simulink model "LQRxSTM"  (R2025b)
settings: Solver=FixedStepDiscrete  StartTime=0.0  StopTime=inf  FixedStep=0.005  RelTol=1e-3
settings Model: Creator=mwali  LastModifiedBy=hassa
settings OptimizationCC: DefaultParameterBehavior=Inlined  UseDivisionForNetSlopeComputation=on  GainParamInheritBuiltInType=on  UseFloatMulNetSlope=on  InlineInvariantSignals=on  PassReuseOutputArgsAs=Individual arguments  ZeroExternalMemoryAtStartup=off  ZeroInternalMemoryAtStartup=off  NoFixptDivByZeroProtection=on  EfficientFloat2IntCast=on  LifeSpan=1  MaxStackSize=512  OptimizeBlockOrder=speed  DifferentSizesBufferReuse=on  EfficientTunableParamExpr=on
settings DebuggingCC: ParameterTunabilityLossMsg=error
settings HardwareCC: ProdBitPerPointer=32.0  ProdBitPerSizeT=32.0  ProdBitPerPtrDiffT=32.0  ProdLargestAtomicInteger=Long  ProdLargestAtomicFloat=Double  ProdWordSize=32.0  ProdLongLongMode=on  ProdHWDeviceType=ARM Compatible->ARM Cortex-M
settings SFSimCC: MATLABDynamicMemAlloc=off
settings RTWCC: SystemTargetFile=ert.tlc  HardwareBoard=STM32H7xx Based (Single-core)  TemplateMakefile=ert_default_tmf  Toolchain=GNU Tools for ARM Embedded Processors  Description=Embedded Coder
settings CodeAppCC: ForceParamTrailComments=on  IgnoreCustomStorageClasses=off  OperatorAnnotations=on  SimulinkDataObjDesc=on  SFDataObjDesc=on  CustomSymbolStrGlobalVar=rt$N$M  CustomSymbolStrType=$N$M  CustomSymbolStrFcn=$N$M$F  CustomSymbolStrMacro=$N$M  InsertBlockDesc=on
settings ERTTargetCC: ExtModeTransport=3.0  ExtModeStaticAlloc=on  ExtModeStaticAllocSize=2048.0  ExtModeMexFile=ext_xcp  ExtModeIntrfLevel=Level2 - Open  ERTFilePackagingFormat=CompactWithDataFile  TargetLangStandard=C99 (ISO)  CodeReplacementLibrary=ARM Cortex-M  IncludeMdlTerminateFcn=off  CombineSignalStateStructs=on  SupportAbsoluteTime=off  SupportComplex=off  SupportNonInlinedSFcns=on

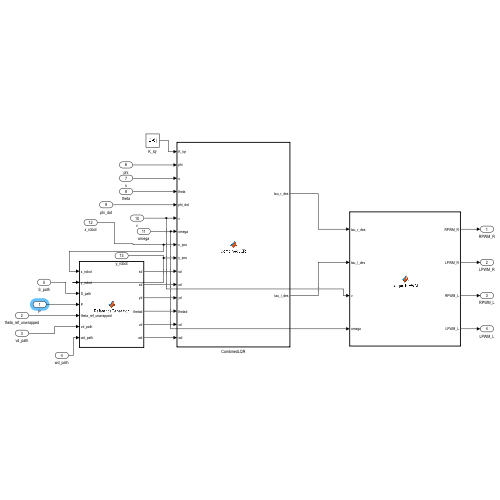
[thumbnail: Simulink's stored preview of the top-level diagram]
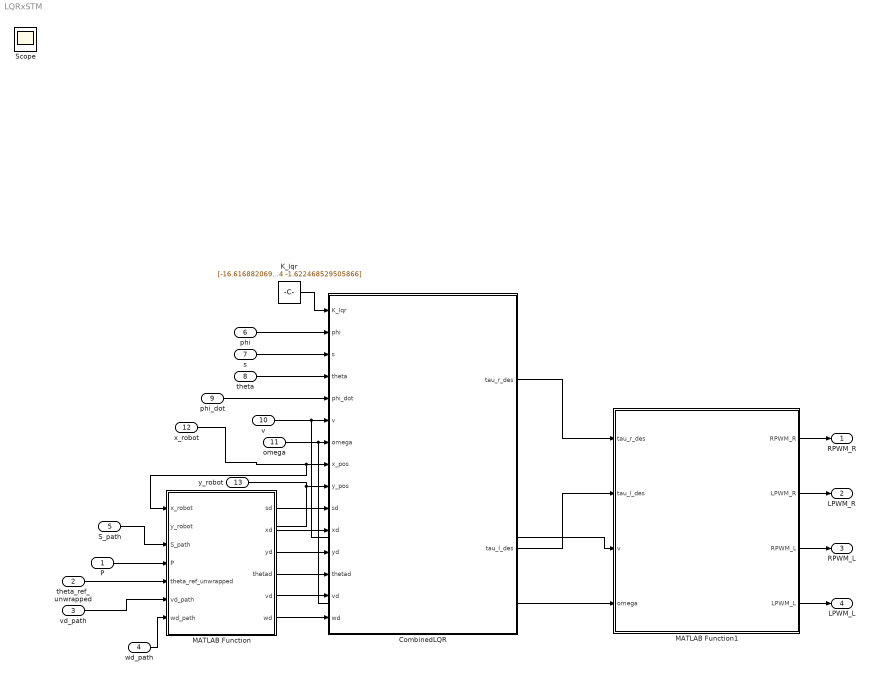
== system LQRxSTM ==
  P : Inport  PortDimensions=[100 2]
  theta_ref_unwrapped : Inport  Port=2  PortDimensions=100
  vd_path : Inport  Port=3  PortDimensions=100
  wd_path : Inport  Port=4  PortDimensions=100
  S_path : Inport  Port=5  PortDimensions=100
  phi : Inport  Port=6
  s : Inport  Port=7
  theta : Inport  Port=8
  phi_dot : Inport  Port=9
  v : Inport  Port=10
  omega : Inport  Port=11
  x_robot : Inport  Port=12
  y_robot : Inport  Port=13
  CombinedLQR : MATLAB Function  TreatAsAtomicUnit=on
  K_lqr : Constant  Value=|
      | [-16.616882069954595	-1.118033988749899	3.162277660168384	-2.938330914554923	-2.061355185548641	1.622468529505869;
      | -16.616882069954599	-1.118033988749900	-3.162277660168376	-2.938330914554922	-2.061355185548644	-1.622468529505866]
  MATLAB Function : MATLAB Function  TreatAsAtomicUnit=on
  MATLAB Function1 : MATLAB Function  TreatAsAtomicUnit=on
  RPWM_R : Outport
  LPWM_R : Outport  Port=2
  RPWM_L : Outport  Port=3
  LPWM_L : Outport  Port=4
  Scope : Scope
      settings: ActiveDisplayYMinimum=-0.34848844243079913  ActiveDisplayYMaximum=2.6945477005962535
  wires:
  MATLAB Function/2(xd) -> CombinedLQR/11(xd)
  phi_dot/1 -> CombinedLQR/5(phi_dot)
  theta/1 -> CombinedLQR/4(theta)
  S_path/1 -> MATLAB Function/3(S_path)
  MATLAB Function/3(yd) -> CombinedLQR/12(yd)
  y_robot/1 -> MATLAB Function/2(y_robot), CombinedLQR/9(y_pos)
  v/1 -> MATLAB Function1/3(v), CombinedLQR/6(v)
  omega/1 -> MATLAB Function1/4(omega), CombinedLQR/7(omega)
  x_robot/1 -> MATLAB Function/1(x_robot), CombinedLQR/8(x_pos)
  s/1 -> CombinedLQR/3(s)
  MATLAB Function1/2(LPWM_R) -> LPWM_R/1
  MATLAB Function1/1(RPWM_R) -> RPWM_R/1
  MATLAB Function/1(sd) -> CombinedLQR/10(sd)
  CombinedLQR/1(tau_r_des) -> MATLAB Function1/1(tau_r_des)
  CombinedLQR/2(tau_l_des) -> MATLAB Function1/2(tau_l_des)
  MATLAB Function/6(wd) -> CombinedLQR/15(wd)
  MATLAB Function/4(thetad) -> CombinedLQR/13(thetad)
  phi/1 -> CombinedLQR/2(phi)
  MATLAB Function/5(vd) -> CombinedLQR/14(vd)
  K_lqr/1 -> CombinedLQR/1(K_lqr)
  MATLAB Function1/3(RPWM_L) -> RPWM_L/1
  MATLAB Function1/4(LPWM_L) -> LPWM_L/1
  P/1 -> MATLAB Function/4(P)
  theta_ref_unwrapped/1 -> MATLAB Function/5(theta_ref_unwrapped)
  vd_path/1 -> MATLAB Function/6(vd_path)
  wd_path/1 -> MATLAB Function/7(wd_path)

== matlab function LQRxSTM/CombinedLQR ==
  settings: updateMethod=DISCRETE
  data: K_lqr input; phi input; s input; theta input; phi_dot input; v input; omega input; x_pos input; y_pos input; sd input; xd input; yd input; thetad input; vd input; wd input; tau_r_des output; tau_l_des output
function [tau_r_des, tau_l_des] = CombinedLQR( ...
    K_lqr, phi, s, theta, phi_dot, v, omega, x_pos, y_pos, ...
    sd, xd, yd, thetad, vd, wd)
%#codegen

% outputs init
tau_r_des  = 0;
tau_l_des  = 0;
ex_out     = 0;
ey_out     = 0;
etheta_out = 0;

% -----------------------------
% 1) Path position error in world frame
% -----------------------------
dx = xd - x_pos;
dy = yd - y_pos;

% -----------------------------
% 2) Error in robot body frame
% ex = forward error
% et = lateral error
% -----------------------------
ex =  cos(theta)*dx + sin(theta)*dy;
ey = -sin(theta)*dx + cos(theta)*dy;

% save for plotting
ex_out = ex;
ey_out = ey;

% -----------------------------
% 3) Heading correction from lateral error
% -----------------------------
k_y = 0.1;                     % tune this if needed
theta_corr_max = deg2rad(20);  % max heading correction

theta_corr = k_y * ey;

if theta_corr > theta_corr_max
    theta_corr = theta_corr_max;
elseif theta_corr < -theta_corr_max
    theta_corr = -theta_corr_max;
end

thetad_corr = thetad + theta_corr;

% -----------------------------
% 4) State error for LQR
% -----------------------------
e = zeros(6,1);
e(1) =phi ;
e(2) = s - sd; 
e(3) = atan2(sin(theta - thetad_corr), cos(theta - thetad_corr));
e(4) = phi_dot;
e(5) = v - vd;
e(6) = omega - wd;

etheta_out = e(3);

% -----------------------------
% 5) LQR control
% -----------------------------
u_des = -K_lqr * e;

tau_r_des = u_des(1);
tau_l_des = u_des(2);

% -----------------------------
% 6) Torque saturation
% -----------------------------
tau_lim = 3; % Changed from 6 to 3

if tau_r_des > tau_lim
    tau_r_des = tau_lim;
elseif tau_r_des < -tau_lim
    tau_r_des = -tau_lim;
end

if tau_l_des > tau_lim
    tau_l_des = tau_lim;
elseif tau_l_des < -tau_lim
    tau_l_des = -tau_lim;
end

== matlab function LQRxSTM/MATLAB Function ==
  data: x_robot input; y_robot input; S_path input; P input; theta_ref_unwrapped input; vd_path input; wd_path input; sd output; xd output; yd output; thetad output; vd output; wd output
function [sd, xd, yd, thetad, vd, wd] = ReferenceGenerator(x_robot, y_robot, S_path, P, theta_ref_unwrapped, vd_path, wd_path)
    N = size(P, 1);

    % 1. Find the nearest discrete node
    min_dist2 = inf;
    k_min = int32(1);
    for k = int32(1) : int32(N)
        dx = P(k, 1) - x_robot;
        dy = P(k, 2) - y_robot;
        d2 = dx*dx + dy*dy;
        if d2 < min_dist2
            min_dist2 = d2;
            k_min = k;
        end
    end

    % 2. Continuous Projection (Fixes the high-frequency torque chattering)
    k_next = min(k_min + int32(1), int32(N));
    k_prev = max(k_min - int32(1), int32(1));

    d2_next = (P(k_next,1)-x_robot)^2 + (P(k_next,2)-y_robot)^2;
    d2_prev = (P(k_prev,1)-x_robot)^2 + (P(k_prev,2)-y_robot)^2;

    if d2_next < d2_prev
        k1 = k_min;
        k2 = k_next;
    else
        k1 = k_prev;
        k2 = k_min;
    end

    if k1 == k2
        alpha = 0.0;
    else
        vx = P(k2,1) - P(k1,1);
        vy = P(k2,2) - P(k1,2);
        L2 = vx*vx + vy*vy;
        if L2 > 1e-6
            rx = x_robot - P(k1,1);
            ry = y_robot - P(k1,2);
            % Orthogonal projection scalar
            alpha = (rx*vx + ry*vy) / L2;
            alpha = max(0.0, min(1.0, alpha));
        else
            alpha = 0.0;
        end
    end

    % 3. Interpolate perfectly smooth references (No Lookahead)
    sd     = (1 - alpha) * S_path(k1) + alpha * S_path(k2);
    xd     = (1 - alpha) * P(k1, 1)   + alpha * P(k2, 1);
    yd     = (1 - alpha) * P(k1, 2)   + alpha * P(k2, 2);
    thetad = (1 - alpha) * theta_ref_unwrapped(k1) + alpha * theta_ref_unwrapped(k2);
    vd     = (1 - alpha) * vd_path(k1) + alpha * vd_path(k2);
    wd     = (1 - alpha) * wd_path(k1) + alpha * wd_path(k2);

    % 4. Safety clamps
    vd_max = 0.3;
    wd_max = 0.334;
    vd = max(0, min(vd, vd_max));
    wd = max(min(wd, wd_max), -wd_max);
end

== matlab function LQRxSTM/MATLAB Function1 ==
  data: tau_r_des input; RPWM_R output; tau_l_des input; v input; omega input; LPWM_R output; RPWM_L output; LPWM_L output
function [RPWM_R, LPWM_R, RPWM_L, LPWM_L] = TorqueToPWM(tau_r_des, tau_l_des, v, omega)
    % --- NFP-42GP-775-EN Motor Parameters ---
    K_t = 0.6746;      % Torque constant (Nm/A)
    K_e = 0.6746;      % Back-EMF constant (V/(rad/s))
    R_res = 0.9796;    % Armature resistance (Ohms)
    V_batt = 24.0;     % Battery voltage (V)
    
    % --- Controller & Robot Parameters ---
    max_pwm = 1000;    % 10-bit timer
    r = 0.060;         % Wheel radius (m)
    d = 0.450;         % Wheelbase (m)
    
    % 1. Estimate wheel speeds (rad/s)
    omega_wheel_r = (v + (omega * d / 2)) / r;
    omega_wheel_l = (v - (omega * d / 2)) / r;

    % 2. Calculate Voltages (V = I*R + Back_EMF)
    v_r = ((tau_r_des / K_t) * R_res) + (K_e * omega_wheel_r);
    v_l = ((tau_l_des / K_t) * R_res) + (K_e * omega_wheel_l);

    % 3. Convert to PWM and Clamp
    pwm_r = round((v_r / V_batt) * max_pwm);
    pwm_l = round((v_l / V_batt) * max_pwm);
    
    % Clamping logic
    pwm_r = max(min(pwm_r, max_pwm), -max_pwm);
    pwm_l = max(min(pwm_l, max_pwm), -max_pwm);

    if pwm_r >= 0
        RPWM_R = pwm_r;
        LPWM_R = 0;
    else
        RPWM_R = 0;
        LPWM_R = abs(pwm_r); 
    end

    if pwm_l >= 0
        RPWM_L = pwm_l;
        LPWM_L = 0;
    else
        RPWM_L = 0;
        LPWM_L = abs(pwm_l); 
    end
end
